simulink model "KF"  (R2021a)
settings: Solver=VariableStepAuto  StartTime=0.0  StopTime=40  RelTol=1e-3
values from neighbouring files (symbols this model uses):
  A = sys_d.A    [KFAlqueva.m]    (also in KFMadeira1.m; KFPortoSanto.m)
  B = sys_d.B    [KFAlqueva.m]    (also in KFMadeira1.m; KFPortoSanto.m)
  bias_init = 0.01    [KFAlqueva.m]    (also in KFMadeira1.m; KFPortoSanto.m)
  C = sys_d.C    [KFAlqueva.m]    (also in KFMadeira1.m; KFPortoSanto.m)
  zsimucorr = [timesimu' zsamp.*cosd(pitch(stg:fg)).*cosd(roll(stg:fg))]    [KFAlqueva.m]    (also in KFMadeira1.m; KFMontargil.m; KFPortoSanto.m = round([timesimu' zsamp.*cosd(pitch(stg:fg)).*cosd(roll(stg:f)
undefined symbols (not defined in the file or in its folder): m
settings Model: Creator=Simão Amaro  LastModifiedBy=simao

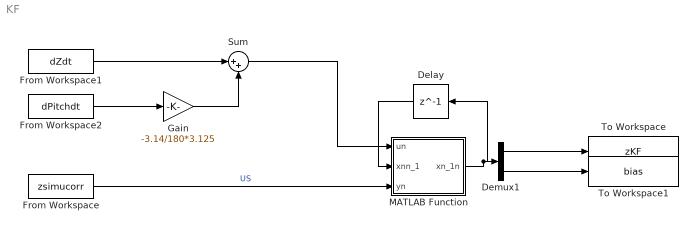
== system KF ==
  Delay : Delay  DelayLength=1  InitialCondition=[round(zsimucorr(1,2),4);bias_init]  SampleTime=0.02
  Demux1 : Demux  Outputs=2
  From Workspace : FromWorkspace  VariableName=zsimucorr  SampleTime=0.02
  From Workspace1 : FromWorkspace  VariableName=dZdt  SampleTime=0.02
  From Workspace2 : FromWorkspace  VariableName=dPitchdt  SampleTime=0.02
  Gain : Gain  Gain=-3.14/180*3.125
  MATLAB Function : MATLAB Function  TreatAsAtomicUnit=on
  Sum : Sum  Inputs=|++
  To Workspace : ToWorkspace  VariableName=zKF  SaveFormat=Timeseries  SampleTime=0.02
  To Workspace1 : ToWorkspace  VariableName=bias  SaveFormat=Timeseries  SampleTime=0.02
  wires:
  From Workspace2/1 -> Gain/1
  From Workspace1/1 -> Sum/1
  MATLAB Function/1(xn_1n) -> Delay/1, Demux1/1
  Delay/1 -> MATLAB Function/2(xnn_1)
  Demux1/1 -> To Workspace/1
  Gain/1 -> Sum/2
  Demux1/2 -> To Workspace1/1
  Sum/1 -> MATLAB Function/1(un)
  From Workspace/1 -> MATLAB Function/3(yn)  "US"

== matlab function KF/MATLAB Function ==
  data: un input; xnn_1 input; yn input; xn_1n output; m parameter; A parameter; B parameter; C parameter
function xn_1n = fcn(un,xnn_1,yn,m, A, B, C)

xnn   = xnn_1 + m*(yn - C*xnn_1);
xn_1n = A*xnn + B*un;
